simulink model "traslacion_carro"  (R2019a)
settings: Solver=VariableStepAuto  StartTime=0.0  StopTime=10.0  RelTol=1e-3
values from neighbouring files (symbols this model uses):
  b_eq_c = 30.0    (= 30)    [parametros.m]
  J_eq_c = m_c + ( J_w + i_c^2*J_m_c ) / R_w^2    (= 59008)    [parametros.m]
  x_0 = -20.0    (= -20)    [parametros.m]
settings Model: Creator=Facundo  LastModifiedBy=Facundo
settings DataIOCC: SaveOutput=off  SaveTime=off

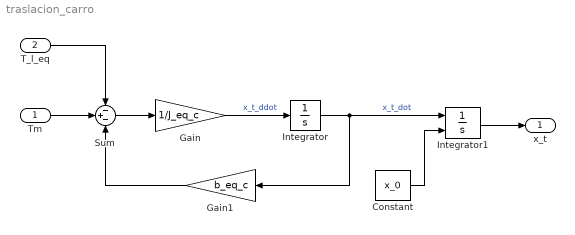
== system traslacion_carro ==
  Tm : Inport  OutDataTypeStr=double  PortDimensions=1  SampleTime=0
  T_l_eq : Inport  Port=2  OutDataTypeStr=double  PortDimensions=1  SampleTime=0
  Constant : Constant  Value=x_0
  Gain : Gain  Gain=1/J_eq_c
  Gain1 : Gain  Gain=b_eq_c
  Integrator : Integrator
  Integrator1 : Integrator  InitialConditionSource=external
  Sum : Sum  Inputs=-+-
  x_t : Outport  OutDataTypeStr=double  PortDimensions=1  SampleTime=0
  wires:
  Gain/1 -> Integrator/1  "x_t_ddot"
  Tm/1 -> Sum/2
  Integrator1/1 -> x_t/1
  Sum/1 -> Gain/1
  Integrator/1 -> Integrator1/1, Gain1/1  "x_t_dot"
  T_l_eq/1 -> Sum/1
  Gain1/1 -> Sum/3
  Constant/1 -> Integrator1/2
